simulink model "circuito_boost"  (R2021b)
settings: Solver=FixedStepAuto  StartTime=0.0  StopTime=0.008  FixedStep=(32e-6)/100  RelTol=1e-3
undefined symbols (not defined in the file or in its folder): C, D, L, Rl, T, Vi
libraries: spsCurrentMeasurementLib x5, spsVoltageMeasurementLib x5, spsSeriesRLCBranchLib x3, spsDiodeLib x1, spsDCVoltageSourceLib x1, spsMosfetLib x1, spsNeutralLib x1, spspowerguiLib x1
settings Model: Creator=hecto  LastModifiedBy=hecto

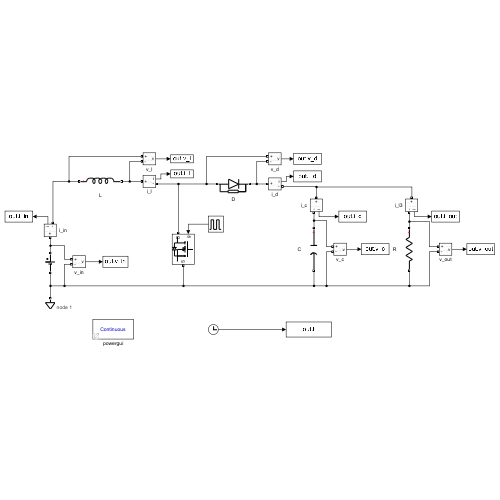
[thumbnail: Simulink's stored preview of the top-level diagram]
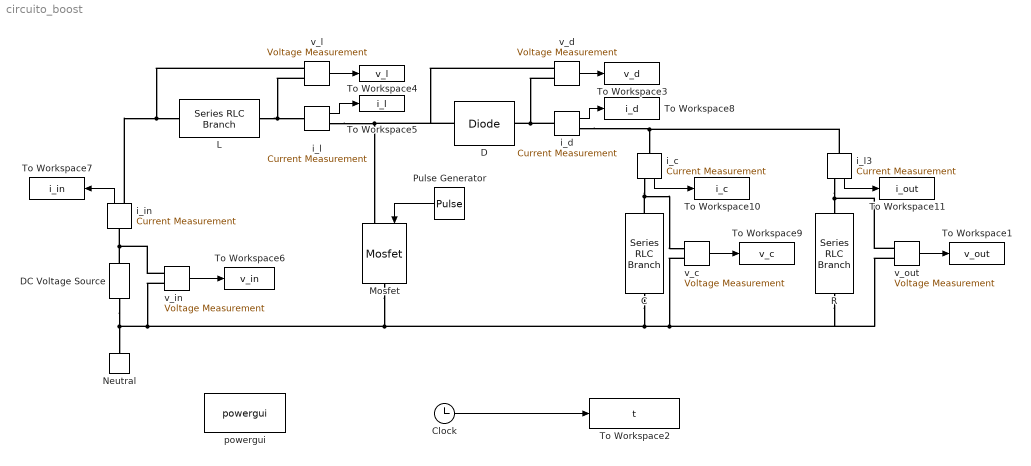
== system circuito_boost ==
  C : spsSeriesRLCBranchLib/Series RLC Branch  LConnTagsString=__new0  RConnTagsString=__new0  BranchType=C  Resistance=0  Inductance=1e-3  SetiL0=off  InitialCurrent=0  Capacitance=C  Setx0=off  InitialVoltage=0  Measurements=None
  Clock : Clock
  D : spsDiodeLib/Diode  Ron=0.001  Lon=0  Vf=0.8  IC=0  UseSnubber=0  Rs=500  Cs=250e-9  Measurements=off
  DC Voltage Source : spsDCVoltageSourceLib/DC Voltage Source  Amplitude=Vi  Measurements=None
  L : spsSeriesRLCBranchLib/Series RLC Branch  LConnTagsString=__new0  RConnTagsString=__new0  BranchType=L  Resistance=0  Inductance=L  SetiL0=off  InitialCurrent=0  Capacitance=0  Setx0=off  InitialVoltage=0  Measurements=None
  Mosfet : spsMosfetLib/Mosfet  Ron=0.1  Lon=0  Rd=0.01  Vfd=0  IC=0  Rs=1e5  Cs=inf  Measurements=off
  Neutral : spsNeutralLib/Neutral  LConnTagsString=a  NodeNumber=1
      settings: AttributesFormatString=node %<NodeNumber>  SourceProductBaseCode=PS
  Pulse Generator : DiscretePulseGenerator  PulseType=Time based  Period=T  PulseWidth=D*100
  R : spsSeriesRLCBranchLib/Series RLC Branch  LConnTagsString=__new0  RConnTagsString=__new0  BranchType=R  Resistance=Rl  Inductance=1e-3  SetiL0=off  InitialCurrent=0  Capacitance=0  Setx0=off  InitialVoltage=0  Measurements=None
  To Workspace1 : ToWorkspace  VariableName=v_out  SampleTime=-1
  To Workspace10 : ToWorkspace  VariableName=i_c  SampleTime=-1
  To Workspace11 : ToWorkspace  VariableName=i_out  SampleTime=-1
  To Workspace2 : ToWorkspace  VariableName=t  SampleTime=-1
  To Workspace3 : ToWorkspace  VariableName=v_d  SampleTime=-1
  To Workspace4 : ToWorkspace  VariableName=v_l  SampleTime=-1
  To Workspace5 : ToWorkspace  VariableName=i_l  SampleTime=-1
  To Workspace6 : ToWorkspace  VariableName=v_in  SampleTime=-1
  To Workspace7 : ToWorkspace  VariableName=i_in  SampleTime=-1
  To Workspace8 : ToWorkspace  VariableName=i_d  SampleTime=-1
  To Workspace9 : ToWorkspace  VariableName=v_c  SampleTime=-1
  i_c : spsCurrentMeasurementLib/Current Measurement  PhasorSimulation=off  OutputType=Complex  PSBequivalent=0
  i_d : spsCurrentMeasurementLib/Current Measurement  PhasorSimulation=off  OutputType=Complex  PSBequivalent=0
  i_in : spsCurrentMeasurementLib/Current Measurement  PhasorSimulation=off  OutputType=Complex  PSBequivalent=0
  i_l : spsCurrentMeasurementLib/Current Measurement  PhasorSimulation=off  OutputType=Complex  PSBequivalent=0
  i_l3 : spsCurrentMeasurementLib/Current Measurement  PhasorSimulation=off  OutputType=Complex  PSBequivalent=0
  powergui : spspowerguiLib/powergui  Priority=1  SimulationMode=Continuous  SampleTime=50e-6  frequency=60  Iterations=50  frequencyindice=0  Pbase=100e6  ErrMax=1e-4  UnitsV=kV  UnitsW=MW  buscounter=0  FunctionMessages=off  echomessages=off  EnableUseOfTLC=off  CurrentSourceSwitches=off  DisableSnubberDevices=off  DisableRonSwitches=off  DisableVfSwitches=off  DisplayEquations=off  AutomaticDiscreteSolvers=off  SolverType=Tustin/Backward Euler (TBE)  Interpol=off  ExternalGateDelay=off  methode=off  Ts=100  x0status=blocks  SPID=on  SwTol=0  HookPort=off  NonlinearTolerance=1e-4  nMaxIteration=100  ContinueOnMaxIteration=off  RestoreLinks=warning  ResistiveCurrentMeasurement=off  Frange=[0:2:500]  Ylog=off  Xlog=on  ShowGrid=off  save=off  variable=ZData  structure=0  ZoomFFT=off  StartTime=0.0  cycles=1  DisplayStyle=1  fundamental=60  FreqAxis=off  MaxFrequency=1000  frequencyindicesteady=1  RmsSteady=1  display=off
  v_c : spsVoltageMeasurementLib/Voltage Measurement  PhasorSimulation=off  OutputType=Complex  PSBequivalent=0
  v_d : spsVoltageMeasurementLib/Voltage Measurement  PhasorSimulation=off  OutputType=Complex  PSBequivalent=0
  v_in : spsVoltageMeasurementLib/Voltage Measurement  PhasorSimulation=off  OutputType=Complex  PSBequivalent=0
  v_l : spsVoltageMeasurementLib/Voltage Measurement  PhasorSimulation=off  OutputType=Complex  PSBequivalent=0
  v_out : spsVoltageMeasurementLib/Voltage Measurement  PhasorSimulation=off  OutputType=Complex  PSBequivalent=0
  wires:
  Pulse Generator/1 -> Mosfet/1
  Clock/1 -> To Workspace2/1
  v_in/1 -> To Workspace6/1
  i_in/1 -> To Workspace7/1
  v_l/1 -> To Workspace4/1
  i_l/1 -> To Workspace5/1
  v_d/1 -> To Workspace3/1
  i_d/1 -> To Workspace8/1
  v_c/1 -> To Workspace9/1
  v_out/1 -> To Workspace1/1
  i_l3/1 -> To Workspace11/1
  i_c/1 -> To Workspace10/1
  connections:
  DC Voltage Source/LConn1 -- R/RConn1 -- v_out/LConn2 -- v_c/LConn2 -- C/RConn1 -- Mosfet/RConn1 -- v_in/LConn2 -- Neutral/LConn1
  DC Voltage Source/RConn1 -- i_in/LConn1 -- v_in/LConn1
  i_in/RConn1 -- v_l/LConn1 -- L/LConn1
  L/RConn1 -- v_l/LConn2 -- i_l/LConn1
  i_l/RConn1 -- v_d/LConn1 -- D/LConn1 -- Mosfet/LConn1
  i_d/LConn1 -- v_d/LConn2 -- D/RConn1
  i_d/RConn1 -- i_l3/LConn1 -- i_c/LConn1
  i_c/RConn1 -- C/LConn1 -- v_c/LConn1
  i_l3/RConn1 -- v_out/LConn1 -- R/LConn1
